simulink model "Generalized_Simulink_Control_System_5_21_18"  (R2018a)
settings: Solver=FixedStepAuto  StartTime=0.0  StopTime=inf  FixedStep=.015  RelTol=1e-3  EnableMultiTasking=on
libraries: raspberrypilib x24, hdlsllib x21, simulink x11
(part 2 of 2)

== system Generalized_Simulink_Control_System_5_21_18/Control System/SSIV Hardware Communication/radio_throttle return message (Slave --> Master) ==
  In1 : Inport
  8 bytes concatinated converted to double : DataTypeConversion  OutDataTypeStr=double  RndMeth=Nearest
  Bit Concat : hdlsllib/Logic and Bit Operations/Bit Concat  numInputs=2
      settings: SourceProductName=HDL Coder  SourceProductBaseCode=HD
  Bytes of the return message : Display
      settings: Format=decimal (Stored Integer)
  Data Type Conversion : DataTypeConversion  OutDataTypeStr=int16  RndMeth=Nearest
  Demux : Demux
  Display : Display
      settings: Format=binary (Stored Integer)
  Display1 : Display
      settings: Format=decimal (Stored Integer)
  Display2 : Display
      settings: Format=binary (Stored Integer)
  radio_throttle : Outport
  wires:
  8 bytes concatinated converted to double/1 -> Display1/1, radio_throttle/1  "radio_throttle"
  Demux/2 -> Display2/1  "Slave Status"
  Demux/1 -> Display/1  "Previous Data"
  In1/1 -> Bytes of the return message/1, Demux/1
  Bit Concat/1 -> Data Type Conversion/1
  Demux/4 -> Bit Concat/1
  Demux/3 -> Bit Concat/2
  Data Type Conversion/1 -> 8 bytes concatinated converted to double/1

== system Generalized_Simulink_Control_System_5_21_18/Control System/SSIV Hardware Communication/servo_out Write Message (Master --> Slave) ==
  In1 : Inport
  Bit Slice2 : hdlsllib/Logic and Bit Operations/Bit Slice  lidx=15  ridx=8
  Bit Slice3 : hdlsllib/Logic and Bit Operations/Bit Slice  lidx=7  ridx=0
  Display5 : Display
      settings: Format=decimal (Stored Integer)
  Mux : Mux  Inputs=2
      settings: DisplayOption=signals
  Out1 : Outport
  wires:
  In1/1 -> Display5/1, Bit Slice3/1, Bit Slice2/1  "Servo"
  Mux/1 -> Out1/1
  Bit Slice3/1 -> Mux/1
  Bit Slice2/1 -> Mux/2

== system Generalized_Simulink_Control_System_5_21_18/Control System/SSIV Hardware Communication/throttle_left_front Write Message (Master --> Slave) ==
  In1 : Inport
  Bit Slice : hdlsllib/Logic and Bit Operations/Bit Slice  lidx=15  ridx=8
  Bit Slice1 : hdlsllib/Logic and Bit Operations/Bit Slice  lidx=7  ridx=0
  Display4 : Display
  Mux : Mux  Inputs=2
      settings: DisplayOption=signals
  Output : Outport
  wires:
  Mux/1 -> Output/1
  Bit Slice/1 -> Display4/1, Mux/2
  Bit Slice1/1 -> Mux/1
  In1/1 -> Bit Slice/1, Bit Slice1/1

== system Generalized_Simulink_Control_System_5_21_18/Control System/SSIV Hardware Communication/throttle_left_rear Write Message (Master --> Slave) ==
  In1 : Inport
  Bit Slice : hdlsllib/Logic and Bit Operations/Bit Slice  lidx=15  ridx=8
  Bit Slice1 : hdlsllib/Logic and Bit Operations/Bit Slice  lidx=7  ridx=0
  Display4 : Display
  Mux : Mux  Inputs=2
      settings: DisplayOption=signals
  Output : Outport
  wires:
  In1/1 -> Bit Slice1/1, Bit Slice/1
  Bit Slice1/1 -> Mux/1
  Bit Slice/1 -> Mux/2, Display4/1
  Mux/1 -> Output/1

== system Generalized_Simulink_Control_System_5_21_18/Control System/SSIV Hardware Communication/throttle_right_front Write Message (Master --> Slave) ==
  In1 : Inport
  Bit Slice : hdlsllib/Logic and Bit Operations/Bit Slice  lidx=15  ridx=8
  Bit Slice1 : hdlsllib/Logic and Bit Operations/Bit Slice  lidx=7  ridx=0
  Display4 : Display
  Mux : Mux  Inputs=2
      settings: DisplayOption=signals
  Output : Outport
  wires:
  Mux/1 -> Output/1
  Bit Slice/1 -> Display4/1, Mux/2
  Bit Slice1/1 -> Mux/1
  In1/1 -> Bit Slice/1, Bit Slice1/1

== system Generalized_Simulink_Control_System_5_21_18/Control System/SSIV Hardware Communication/throttle_right_rear Write Message (Master --> Slave) ==
  In1 : Inport
  Bit Slice : hdlsllib/Logic and Bit Operations/Bit Slice  lidx=15  ridx=8
  Bit Slice1 : hdlsllib/Logic and Bit Operations/Bit Slice  lidx=7  ridx=0
  Display4 : Display
  Mux : Mux  Inputs=2
      settings: DisplayOption=signals
  Output : Outport
  wires:
  In1/1 -> Bit Slice1/1, Bit Slice/1
  Bit Slice1/1 -> Mux/1
  Bit Slice/1 -> Mux/2, Display4/1
  Mux/1 -> Output/1
